simulink model "Gesamtsystem_Prototyp25_01_3"  (R2021b)
settings: Solver=FixedStepDiscrete  StartTime=0.0  StopTime=Inf  RelTol=1e-3  EnableMultiTasking=on
undefined symbols (not defined in the file): Down, GPTRIP1SEL, GPTRIP2SEL, magnitude, TZ1, TZ2, Up
libraries: c2837xDlib x18, hdlsllib x10, simulink x5, c2802xlib x5, c280xlib x3, dspsigops x3, commsequence2 x2, idelinklib_common x2, mcbcontrolslib x2, c2000lib x1, dspstat3 x1
(part 3 of 3)

== system Gesamtsystem_Prototyp25_01_3/Kommunikation/I2C Receiver/DecodeNexonar/Subsystem2 ==
  packed : Inport
  Bit Shift : hdlsllib/Logic and Bit Operations/Bit Shift  mode=Shift Left Logical  N=8
  Data Type Conversion : DataTypeConversion  OutDataTypeStr=int16
  Demux : Demux  Outputs=2
  Sum : Sum  Inputs=|++
  unpacked : Outport
  wires:
  packed/1 -> Demux/1
  Sum/1 -> Data Type Conversion/1
  Demux/1 -> Bit Shift/1
  Bit Shift/1 -> Sum/1
  Demux/2 -> Sum/2
  Data Type Conversion/1 -> unpacked/1

== system Gesamtsystem_Prototyp25_01_3/Kommunikation/I2C Receiver/DecodeNexonar/Subsystem3 ==
  packed : Inport
  Bit Shift : hdlsllib/Logic and Bit Operations/Bit Shift  mode=Shift Left Logical  N=8
  Data Type Conversion : DataTypeConversion  OutDataTypeStr=int16
  Demux : Demux  Outputs=2
  Sum : Sum  Inputs=|++
  unpacked : Outport
  wires:
  Data Type Conversion/1 -> unpacked/1
  Demux/2 -> Sum/2
  Bit Shift/1 -> Sum/1
  Demux/1 -> Bit Shift/1
  Sum/1 -> Data Type Conversion/1
  packed/1 -> Demux/1

== system Gesamtsystem_Prototyp25_01_3/Navigation und Uebergabe/Steuerung Fahrzeug/PWM/Drossel fuer Rueckwaertsfahren ==
  pwm_out_strecke : Inport
  rueckwaerts : Inport  Port=2
  Gain : Gain  Gain=0.8
  Switch : Switch  Criteria=u2 > Threshold
  Out1 : Outport
  wires:
  Gain/1 -> Switch/3
  rueckwaerts/1 -> Switch/2
  Switch/1 -> Out1/1
  pwm_out_strecke/1 -> Switch/1, Gain/1

== system Gesamtsystem_Prototyp25_01_3/Navigation und Uebergabe/Steuerung Fahrzeug/PWM/Drossel fuer Rueckwaertsfahren1 ==
  pwm_out_strecke : Inport
  rueckwaerts : Inport  Port=2
  Gain : Gain  Gain=0.8
  Switch : Switch  Criteria=u2 > Threshold
  Out1 : Outport
  wires:
  Gain/1 -> Switch/3
  rueckwaerts/1 -> Switch/2
  Switch/1 -> Out1/1
  pwm_out_strecke/1 -> Switch/1, Gain/1

== system Gesamtsystem_Prototyp25_01_3/Navigation und Uebergabe/Steuerung Fahrzeug/PWM/Inverter ==
  In1 : Inport
  Constant2 : Constant  Value=0
  Constant3 : Constant
  Switch : Switch  Criteria=u2 > Threshold  Threshold=0.5
  Out1 : Outport
  wires:
  Constant2/1 -> Switch/1
  Constant3/1 -> Switch/3
  In1/1 -> Switch/2
  Switch/1 -> Out1/1

== system Gesamtsystem_Prototyp25_01_3/Navigation und Uebergabe/Steuerung Fahrzeug/PWM/P-Regler mit Regelfehler Begrenzung Initial: k = 0.1, limit = +//- 100 Sampletime 0.1 ==
  a_soll : Inport
  a_ist : Inport  Port=2
  Abs : Abs  SampleTime=0.01
  Begrenzung : Saturate  UpperLimit=40  LowerLimit=0
  Betrag : MATLAB Function  TreatAsAtomicUnit=on  SystemSampleTime=0.01
  Dead Zone : DeadZone  LowerValue=-5  UpperValue=5  SaturateOnIntegerOverflow=on
  Richtung : MATLAB Function  TreatAsAtomicUnit=on  SystemSampleTime=0.01
  Sum : Sum  Inputs=|-+  SampleTime=0.01
  Verstaerkung : Gain  SampleTime=0.01
  pwm_out_a : Outport  VectorParamsAs1DForOutWhenUnconnected=off
  r/l_out_a : Outport  Port=2  VectorParamsAs1DForOutWhenUnconnected=off
  wires:
  Betrag/1(y) -> pwm_out_a/1
  Verstaerkung/1 -> Abs/1, Richtung/1(u)
  Sum/1 -> Dead Zone/1
  Abs/1 -> Begrenzung/1
  a_soll/1 -> Sum/2
  Richtung/1(y) -> r/l_out_a/1
  a_ist/1 -> Sum/1
  Begrenzung/1 -> Betrag/1(u)
  Dead Zone/1 -> Verstaerkung/1

== system Gesamtsystem_Prototyp25_01_3/Navigation und Uebergabe/Steuerung Fahrzeug/PWM/P-Regler mit Regelfehler Begrenzung Initial: k = 0.1, limit = +//- 100 Sampletime 0.2 ==
  strecke_ist : Inport
  strecke_soll : Inport  Port=2
  Abs : Abs  SampleTime=0.01
  Begrenzung : Saturate  UpperLimit=60  LowerLimit=0
  Betrag : MATLAB Function  TreatAsAtomicUnit=on  SystemSampleTime=0.01
  Dead Zone : DeadZone  SaturateOnIntegerOverflow=on
  Richtung : MATLAB Function  TreatAsAtomicUnit=on  SystemSampleTime=0.01
  Sum : Sum  Inputs=|-+  SampleTime=0.01
  Verstaerkung : Gain  Gain=1.5  SampleTime=0.01
  pwm_out_strecke : Outport  VectorParamsAs1DForOutWhenUnconnected=off
  r/l_out_strecke : Outport  Port=2  VectorParamsAs1DForOutWhenUnconnected=off
  wires:
  Betrag/1(y) -> pwm_out_strecke/1
  Verstaerkung/1 -> Abs/1, Richtung/1(u)
  Sum/1 -> Dead Zone/1
  Abs/1 -> Begrenzung/1
  strecke_soll/1 -> Sum/2
  Richtung/1(y) -> r/l_out_strecke/1
  strecke_ist/1 -> Sum/1
  Begrenzung/1 -> Betrag/1(u)
  Dead Zone/1 -> Verstaerkung/1

== matlab function Gesamtsystem_Prototyp25_01_3/Navigation und Uebergabe/Steuerung Fahrzeug/PWM/P-Regler mit Regelfehler Begrenzung Initial: k = 0.1, limit = +//- 100 Sampletime 0.1/Betrag ==
  settings: updateMethod=DISCRETE  sampleTime=0.01
  data: u input; y output
function y = fcn( u )

if u > 0.5
    y = u;
else
    y = 0;
end

== matlab function Gesamtsystem_Prototyp25_01_3/Navigation und Uebergabe/Steuerung Fahrzeug/PWM/P-Regler mit Regelfehler Begrenzung Initial: k = 0.1, limit = +//- 100 Sampletime 0.1/Richtung ==
  settings: updateMethod=DISCRETE  sampleTime=0.01
  data: u input; y output
function y = fcn( u )

if u > 0
    y = 1;
else
    y = 0;
end

== stateflow chart Gesamtsystem_Prototyp25_01_3/Navigation und Uebergabe/Steuerung Fahrzeug/PWM/Richtungsvorgabe links ==
  state Richtung_R
    r_l_out = r_l_out_strecke
  state Richtung_L
    r_l_out = r_l_out_a;
  (default) -> Richtung_R
  Richtung_R -> Richtung_L : [pwm_out_strecke < pwm_out_a]
  Richtung_L -> Richtung_R : [pwm_out_strecke >= pwm_out_a]
  data: r_l_out_strecke input; r_l_out_a input; pwm_out_strecke input; pwm_out_a input; r_l_out output

== stateflow chart Gesamtsystem_Prototyp25_01_3/Navigation und Uebergabe/Steuerung Fahrzeug/PWM/Stärke PWM L//R ==
  state a
    pwm_res_r = pwm_out_strecke + pwm_out_a;
    pwm_res_l = abs(pwm_out_strecke - pwm_out_a);
  state a1
    pwm_res_r = abs(pwm_out_strecke - pwm_out_a);
    pwm_res_l = pwm_out_strecke + pwm_out_a;
  (default) -> a
  a -> a1 : [r_l_out_a ~= r_l_out_strecke]
  a1 -> a : [r_l_out_a == r_l_out_strecke]
  data: r_l_out_a input; pwm_res_l output; r_l_out_strecke input; pwm_out_strecke input; pwm_out_a input; pwm_res_r output

== stateflow chart Gesamtsystem_Prototyp25_01_3/Navigation und Uebergabe/Steuerung Fahrzeug/PWM/Richtungsvorgabe rechts ==
  state Richtung_R
    r_l_out = r_l_out_strecke;
  state Richtung_L
    r_l_out = r_l_out_a;
  (default) -> Richtung_R
  Richtung_R -> Richtung_L : [pwm_out_strecke < pwm_out_a]
  Richtung_L -> Richtung_R : [pwm_out_strecke >= pwm_out_a]
  data: r_l_out_strecke input; r_l_out_a input; pwm_out_strecke input; pwm_out_a input; r_l_out output

== matlab function Gesamtsystem_Prototyp25_01_3/Navigation und Uebergabe/Steuerung Fahrzeug/PWM/P-Regler mit Regelfehler Begrenzung Initial: k = 0.1, limit = +//- 100 Sampletime 0.2/Betrag ==
  settings: updateMethod=DISCRETE  sampleTime=0.01
  data: u input; y output
function y = fcn( u )

if u > 0.5
    y = u;
else
    y = 0;
end

== matlab function Gesamtsystem_Prototyp25_01_3/Navigation und Uebergabe/Steuerung Fahrzeug/PWM/P-Regler mit Regelfehler Begrenzung Initial: k = 0.1, limit = +//- 100 Sampletime 0.2/Richtung ==
  settings: updateMethod=DISCRETE  sampleTime=0.01
  data: u input; y output
function y = fcn( u )

if u > 0
    y = 1;
else
    y = 0;
end

== matlab function Gesamtsystem_Prototyp25_01_3/Navigation und Uebergabe/Abwurf und Uebergabe/P-Regler mit Regelfehler Begrenzung Initial: k = 0.1, limit = +//- 100 Sampletime 0.1/Betrag ==
  settings: updateMethod=DISCRETE  sampleTime=0.01
  data: u input; y output
function y = fcn( u )

if u > 0.5
    y = u;
else
    y = 0;
end

== matlab function Gesamtsystem_Prototyp25_01_3/Navigation und Uebergabe/Abwurf und Uebergabe/P-Regler mit Regelfehler Begrenzung Initial: k = 0.1, limit = +//- 100 Sampletime 0.1/Richtung ==
  settings: updateMethod=DISCRETE  sampleTime=0.01
  data: u input; y output
function y = fcn( u )

if u > 0
    y = 1;
else
    y = 0;
end

== matlab function Gesamtsystem_Prototyp25_01_3/Navigation und Uebergabe/Abwurf und Uebergabe/P-Regler mit Regelfehler Begrenzung Initial: k = 0.1, limit = +//- 100 Sampletime 0.2/Betrag ==
  settings: updateMethod=DISCRETE  sampleTime=0.01
  data: u input; y output
function y = fcn( u )

if u > 0.5
    y = u;
else
    y = 0;
end

== matlab function Gesamtsystem_Prototyp25_01_3/Navigation und Uebergabe/Abwurf und Uebergabe/P-Regler mit Regelfehler Begrenzung Initial: k = 0.1, limit = +//- 100 Sampletime 0.2/Richtung ==
  settings: updateMethod=DISCRETE  sampleTime=0.01
  data: u input; y output
function y = fcn( u )

if u > 0
    y = 1;
else
    y = 0;
end

== stateflow chart Gesamtsystem_Prototyp25_01_3/Navigation und Uebergabe/Abwurf und Uebergabe/Abgabe_S_R_B ==
  state Abwurf_S
    y_soll_s = 100;
  state Stillstand
    y_ist_s = 0;
    y_ist_rb = 0;
    y_soll_rb = 0;
    y_soll_s = 0;
  state Abgabe_R_B
    y_soll_rb = 100;
    y_ist_rb = 100 - rb_dir*100;
  (default) -> Stillstand
  Stillstand -> Abgabe_R_B [order 1] : [rb == 1]
  Abwurf_S -> Stillstand : [s==0]
  Abgabe_R_B -> Stillstand : [rb == 0]
  Stillstand -> Abwurf_S [order 2] : [s==1]
  data: y_soll_rb output; y_ist_s output; y_ist_rb output; y_soll_s output; rb input; s input; rb_dir input

== stateflow chart Gesamtsystem_Prototyp25_01_3/Datenuebertragung zu stehendem System/Board Communication ==
  state Start
    n_rot = r;
    n_blau = b;
    andocken = 0;
    abdocken = 0;
    fin = 0;
    a = 0;
  state Andocking
    andocken = 1;
    abdocken = 0;
    a = 1;
  state Angedockt
  state Uebaergabe
    n_rot = r;
    n_blau = b;
    andocken = 1;
    abdocken = 0;
    a = 2;
  state Abdocken
    andocken = 0;
    abdocken = 1;
    a = 3;
  (default) -> Start
  Start -> Start [order 2] : after(0.5, sec)
  Uebaergabe -> Abdocken [order 1] : [zustand == 3]
  Angedockt -> Uebaergabe [order 2] : [zustand == 2]
  Start -> Andocking [order 1] : [zustand == 1]
  Andocking -> Angedockt : [andock == true ]
  Uebaergabe -> Abdocken [order 2] : after(15, sec)
  Angedockt -> Uebaergabe [order 1] : after(15, sec)
  data: n_rot output uint16; a output; andocken output; abdocken output; n_blau output uint16; fin output; b input uint16; r input uint16; zustand input; andock input

== stateflow chart Gesamtsystem_Prototyp25_01_3/Sortierung/Entscheidungen je nach Block ==
  state Roter_Block
    rot = 1;
    blau = 0;
    schwarz = 0;
  state Spannungsparameter_Berechnen
    grenze_rb = (u_rot + u_blau)/2;
    grenze_bs = (u_blau + u_schwarz)/2;
    rot_oben = grenze_rb -(u_blau - u_rot)/4;
    blau_unten = grenze_rb +(u_blau - u_rot)/4;
    blau_oben = grenze_bs - (u_schwarz - u_blau)/4;
    schwarz_unten = grenze_bs + (u_schwarz - u_blau)/4;
    init_farbe = 1;
    led_gruen = 0;
  state Roter_block
    u_rot = U_digital;
    led_rot = 0;
    led_gruen = 1;
  state blauer_block
    u_blau = U_digital;
  state schwarzer_block
    u_schwarz = U_digital;
  state Kontrollpunkt
    init_farbe = 0;
  state Zweites_Eingangsspannung
    U_in_2 = U_digital;
    block_2 = farbe(U_in_2, rot_oben, blau_unten, blau_oben, schwarz_unten);
  state Blauer_Block
    rot = 0;
    blau = 1;
    schwarz = 0;
  state grueneLED_zeichen
    led_gruen = 1;
  state grueneLED_zeichen1
    led_gruen = 0;
  state grueneLED_zeichen2
    led_gruen = 1;
  state Erstes_Eingangssignal
    U_in_1 = U_digital;
    block_1 = farbe(U_in_1, rot_oben, blau_unten, blau_oben, schwarz_unten);
  state Schwarzer_Block
    rot = 0;
    blau = 0;
    schwarz = 1;
  state Init_fehlgeschlagen
    led_rot = 1;
  Roter_Block -> Erstes_Eingangssignal : [U_digital >= 0.6]
  Zweites_Eingangsspannung -> Roter_Block [order 1] : [block_1 == 0 && block_2 == 0]
  Zweites_Eingangsspannung -> Erstes_Eingangssignal [order 4] : [block_1 ~= block_2]
  (default) -> Roter_block
  Kontrollpunkt -> Spannungsparameter_Berechnen [order 1] : [u_rot < u_blau && u_blau < u_schwarz]
  schwarzer_block -> Kontrollpunkt : [trigger3 == 1]
  Roter_block -> blauer_block : [trigger1 == 1]
  blauer_block -> schwarzer_block : [trigger2 == 1]
  Erstes_Eingangssignal -> Zweites_Eingangsspannung [order 1] : after(0.2, sec)
  grueneLED_zeichen1 -> grueneLED_zeichen2 : after(0.5, sec)
  grueneLED_zeichen2 -> Erstes_Eingangssignal : [bereit == 1]
  Zweites_Eingangsspannung -> Blauer_Block [order 2] : [block_1 ==1 && block_2 ==1]
  Spannungsparameter_Berechnen -> grueneLED_zeichen : after(0.5, sec)
  grueneLED_zeichen -> grueneLED_zeichen1 : after(0.5, sec)
  Blauer_Block -> Erstes_Eingangssignal : [U_digital <= 1.3 || U_digital >= 1.9]
  Kontrollpunkt -> Init_fehlgeschlagen [order 2] : [u_rot >= u_blau || u_blau >= u_schwarz || u_rot >= u_schwarz]
  Erstes_Eingangssignal -> Init_fehlgeschlagen [order 2] : [fertig_sortiert == 1]
  Schwarzer_Block -> Erstes_Eingangssignal : [U_digital < 2.0 || U_digital >= 2.6]
  Zweites_Eingangsspannung -> Erstes_Eingangssignal [order 5] : [block_1 == 3 || block_2 == 3]
  Zweites_Eingangsspannung -> Init_fehlgeschlagen [order 6] : [fertig_sortiert == 1]
  Zweites_Eingangsspannung -> Schwarzer_Block [order 3] : [block_1 == 2 && block_2 == 2]
  Init_fehlgeschlagen -> Roter_block : after(1, sec)
  data: U function_input; block function_output; rot_o function_input; blau_u function_input; blau_o function_input; schwarz_u function_input; fertig_sortiert input; led_gruen output; trigger1 input; trigger3 input; trigger2 input; led_rot output; bereit input; rot output; schwarz output; blau output; U_digital input; U_in local; U_in_2 local; block_2 local; block_1 local; U_in_1 local; init_farbe output; init_arr local; init_array local; u_blau local; u_schwarz local; u_rot local; grenze_bs local; grenze_rb local; rot_oben local; blau_unten local; blau_oben local; schwarz_unten local
  function block = farbe(U, rot_o, blau_u, blau_o, schwarz_u):
    | function block = farbe(U, rot_o, blau_u, blau_o, schwarz_u)
    |  if U < rot_o
    |      block = 0;
    |  elseif U > blau_u && U < blau_o
    |      block = 1;
    |  elseif U > schwarz_u && U < 3.0
    |      block = 2;
    |  else 
    |      block = 3;
    |  end

== stateflow chart Gesamtsystem_Prototyp25_01_3/Sortierung/Sortierscheibe/Auslenkung des Sortierrades ==
  state Grundzustand6
    n_rot = n_rot;
    schwarz  =1;
    rot = 0; duty = 1;
  state Grundzustand
    n_rot = i + 1;
    schwarz = 0;
    rot = 1; duty = 1;
  state Grundzustand3
    n_blau = j + 1;
  state Vorgaenger_blau
    auslenkung_soll = auslenkung_aktuell + 70;
  state drehen_entgegengesetzt1
    auslenkung_soll = auslenkung_aktuell - 70;
  state Vorgaenger_blau1
    auslenkung_soll = auslenkung_aktuell + 70;
  state Vorgaenger_rot_schwarz1
    auslenkung_soll = auslenkung_aktuell - 70;
  state Vorgaenger_rot_schwarz
    auslenkung_soll = auslenkung_aktuell - 70;
  state drehen_entgegengesetzt7
    auslenkung_soll = auslenkung_aktuell - 70;
  state drehen_entgegengesetzt8
    auslenkung_soll = auslenkung_aktuell + 70;
  state drehen_entgegengesetzt
    auslenkung_soll = auslenkung_aktuell + 70;
  state Warten2
    auslenkung_soll = auslenkung_ist;
    duty = 0;
  state Warten1
    auslenkung_soll = auslenkung_ist
    auslenkung_aktuell = auslenkung_ist;
  state Warten3
    auslenkung_soll = auslenkung_ist;
  state drehen_entgegengesetzt6
    auslenkung_soll = auslenkung_aktuell - 70;
  state Warten6
    auslenkung_soll = auslenkung_ist;
  state Auslenkung_blau
    auslenkung_soll = auslenkung_aktuell-70;
    j = n_blau; rs = 0; b = 1;
  state drehen_entgegengesetzt3
    auslenkung_soll = auslenkung_aktuell + 70;
  state Auslenkung_rotschwarz_vorgaenger1
    auslenkung_soll = auslenkung_aktuell+70;
    duty = 0; i = n_rot; rs = 1; b = 0;
  state Grundzustand2
    auslenkung_soll = auslenkung_aktuell-70;
    n_blau = 1;
  state Warten
    auslenkung_soll = auslenkung_ist;
    auslenkung_aktuell = auslenkung_ist;
  state drehen_entgegengesetzt2
    auslenkung_soll = auslenkung_aktuell + 70;
  state Grundzustand5
    auslenkung_soll = auslenkung_aktuell-70;
    n_rot = 0;
    schwarz = 1; duty = 1;
  state Grundzustand1
    auslenkung_soll = auslenkung_aktuell-70;
    n_rot = 1;
    rot = 1; duty = 1;
  state drehen_entgegengesetzt5
    auslenkung_soll = auslenkung_aktuell + 70;
  state drehen_entgegengesetzt4
    auslenkung_soll = auslenkung_aktuell + 70;
  state Warten5
    auslenkung_soll = auslenkung_ist;
    rs = 1; b = 0;
  state Warten4
    auslenkung_soll = auslenkung_ist;
    auslenkung_aktuell = auslenkung_ist;
  state Anfangsauslenkung
    auslenkung_soll = 140;
  state Warten_Start
    auslenkung_soll = 70;
    n_blau = 0; n_rot = 0;
    rot = 0; schwarz = 0; duty = 0;
  state Warten7
    auslenkung_soll = auslenkung_ist;
  state Stillstand
    auslenkung_soll = 0;
    duty = 0;
    n_blau = 0; n_rot = 0;
    schwarz = 0; rot = 0;
  Warten3 -> Grundzustand6 [order 3] : [Block_angekommen == 0 && blau == 0 && pos == 1]
  Warten3 -> Grundzustand3 [order 2] : [Block_angekommen == 0 && blau== 1]
  Warten3 -> Grundzustand [order 1] : [Block_angekommen == 0 && blau == 0 && pos == 0]
  Grundzustand -> Vorgaenger_blau1 [order 2] : [b == 1]
  Grundzustand -> Vorgaenger_rot_schwarz1 [order 1] : [rs == 1]
  Grundzustand6 -> Vorgaenger_blau1 [order 2] : [b == 1]
  Grundzustand6 -> Vorgaenger_rot_schwarz1 [order 1] : [rs == 1]
  Grundzustand3 -> Vorgaenger_rot_schwarz [order 1] : [rs == 1]
  Grundzustand3 -> Vorgaenger_blau [order 2] : [b == 1]
  Vorgaenger_blau -> drehen_entgegengesetzt1 [order 2] : after(1, sec)
  Vorgaenger_blau1 -> drehen_entgegengesetzt7 [order 2] : after(1, sec)
  drehen_entgegengesetzt8 -> Vorgaenger_rot_schwarz1 : [after(0.3, sec) || sortierscheibe_trigger == 0]
  drehen_entgegengesetzt -> Vorgaenger_rot_schwarz : [after(0.3, sec) || sortierscheibe_trigger == 0]
  Vorgaenger_rot_schwarz1 -> drehen_entgegengesetzt8 [order 2] : after(1, sec)
  drehen_entgegengesetzt1 -> Vorgaenger_blau : [after(0.3, sec) || sortierscheibe_trigger == 0]
  drehen_entgegengesetzt7 -> Vorgaenger_blau1 : [after(0.3, sec) || sortierscheibe_trigger == 0]
  Vorgaenger_rot_schwarz -> drehen_entgegengesetzt [order 2] : after(1, sec)
  Vorgaenger_blau -> Warten1 [order 1] : [abs(auslenkung_soll -auslenkung_ist) <5 && sortierscheibe_trigger == 0]
  Vorgaenger_rot_schwarz -> Warten1 [order 1] : [abs(auslenkung_soll -auslenkung_ist) <5 && sortierscheibe_trigger == 0]
  Vorgaenger_blau1 -> Warten2 [order 1] : [abs(auslenkung_soll -auslenkung_ist) <5 && sortierscheibe_trigger == 0]
  Vorgaenger_rot_schwarz1 -> Warten2 [order 1] : [abs(auslenkung_soll -auslenkung_ist) <5 && sortierscheibe_trigger == 0]
  Grundzustand1 -> Warten2 [order 1] : [abs(auslenkung_soll - auslenkung_ist) < 5 && sortierscheibe_trigger == 0]
  Grundzustand5 -> Warten2 [order 1] : [abs(auslenkung_soll - auslenkung_ist) < 5 && sortierscheibe_trigger == 0]
  Warten2 -> Auslenkung_rotschwarz_vorgaenger1 : after(0.75, sec)
  Grundzustand2 -> Warten1 [order 1] : [abs(auslenkung_soll - auslenkung_ist) < 5 && sortierscheibe_trigger == 0]
  Warten1 -> Auslenkung_blau : after(0.75, sec)
  Warten6 -> Warten3 : after(1, sec)
  drehen_entgegengesetzt6 -> Auslenkung_rotschwarz_vorgaenger1 : [after(0.3, sec) || sortierscheibe_trigger == 0]
  Auslenkung_rotschwarz_vorgaenger1 -> drehen_entgegengesetzt6 [order 2] : after(1, sec)
  Auslenkung_blau -> drehen_entgegengesetzt3 [order 2] : after(1, sec)
  drehen_entgegengesetzt3 -> Auslenkung_blau : [after(0.3, sec) || sortierscheibe_trigger == 0]
  Auslenkung_blau -> Warten [order 1] : [abs(auslenkung_soll - auslenkung_ist) < 5 && sortierscheibe_trigger == 0]
  Warten -> Warten6 : [Block_angekommen ==0]
  Auslenkung_rotschwarz_vorgaenger1 -> Warten [order 1] : [abs(auslenkung_soll - auslenkung_ist) < 5 && sortierscheibe_trigger == 0]
  drehen_entgegengesetzt2 -> Grundzustand2 : [after(0.3, sec) || sortierscheibe_trigger == 0]
  drehen_entgegengesetzt5 -> Grundzustand1 : [after(0.3, sec) || sortierscheibe_trigger == 0]
  Grundzustand5 -> drehen_entgegengesetzt4 [order 2] : after(1, sec)
  Grundzustand2 -> drehen_entgegengesetzt2 [order 2] : after(1, sec)
  Grundzustand1 -> drehen_entgegengesetzt5 [order 2] : after(1, sec)
  drehen_entgegengesetzt4 -> Grundzustand5 : [after(0.3, sec) || sortierscheibe_trigger == 0]
  Warten5 -> Grundzustand2 [order 1] : [Block_angekommen == 0 && blau== 1]
  Warten5 -> Grundzustand5 [order 3] : [Block_angekommen == 0 && blau == 0 && pos == 1]
  Warten5 -> Grundzustand1 [order 2] : [Block_angekommen == 0 && blau == 0 && pos == 0]
  Warten4 -> Warten5 : after(2, sec)
  Anfangsauslenkung -> Warten4 : [Block_angekommen == 0]
  Warten_Start -> Anfangsauslenkung : after(7, sec)
  Warten7 -> Warten_Start : after(4, sec)
  Stillstand -> Warten7 : [init_farbe == 1]
  (default) -> Stillstand
  data: sortierscheibe_trigger input; n_rot output uint16; duty output; rot output; n_blau output uint16; auslenkung_soll output; Block_angekommen input; auslenkung_ist input; blau input; pos input; i local uint16; j local uint16; schwarz output; init_farbe input; auslenkung_aktuell local; rs local; b local

== matlab function Gesamtsystem_Prototyp25_01_3/Sortierung/Sortierscheibe/P-Regler mit Regelfehler Begrenzung Initial: k = 0.1, limit = +//- 100 Sampletime 0.1/Betrag ==
  settings: updateMethod=DISCRETE  sampleTime=0.01
  data: u input; y output
function y = fcn( u )

if u > 0.5
    y = u;
else
    y = 0;
end

== matlab function Gesamtsystem_Prototyp25_01_3/Sortierung/Sortierscheibe/P-Regler mit Regelfehler Begrenzung Initial: k = 0.1, limit = +//- 100 Sampletime 0.1/Richtung ==
  settings: updateMethod=DISCRETE  sampleTime=0.01
  data: u input; y output
function y = fcn( u )

if u > 0
    y = 1;
else
    y = 0;
end

== stateflow chart Gesamtsystem_Prototyp25_01_3/Sortierung/Weiche/Motor Weiche steuerung ==
  note: pos ist 0 wenn auf rot gestellt
  state Bewegung_nach_rot
    pos=0;
  state Bewegung_nach_blau
    pos=1;
  (default) -> Bewegung_nach_rot
  Bewegung_nach_blau -> Bewegung_nach_rot : [work == 1 && rot == 1 && schwarz == 0]
  Bewegung_nach_rot -> Bewegung_nach_blau : [work == 1 && rot == 0 && schwarz == 1]
  data: rot input; schwarz input; work input; pos output

== matlab function Gesamtsystem_Prototyp25_01_3/Kommunikation/I2C Reset (behebt Stabilitätsprobleme der I2C-Verbindung)/I2C Reset/I2C Reset ==
function fcn()
%#codegen

coder.ceval( 'reset_i2c' );

== stateflow chart Gesamtsystem_Prototyp25_01_3/Sortierung/Weiche/Motor Weiche steuerung1 ==
  state Startausrichtung
    y_soll= y_start;
    y_soll_n = 0;
    pos = 0;
  note: pos ist 0 wenn auf rot gestellt
  state Bewegung_nach_rot
    y_soll =0;
    y_soll_n = y_rot;
    pos = 0;
  state Bereit
    y_soll = 0;
    y_soll_n = 0;
  state Bewegung_nach_schwarz
    y_soll = y_blau;
    y_soll_n = 0;
    pos = 1;
  state Warten
    y_soll = 0;
    y_soll_n = 0;
  state Warten1
    y_soll = 0;
    y_soll_n = 0;
  (default) -> Startausrichtung
  Startausrichtung -> Bereit : after(0.5, sec)
  Bereit -> Bewegung_nach_schwarz [order 2] : [duty == 1 && schwarz == 1 && rot == 0 && pos == 0]
  Bereit -> Bewegung_nach_rot [order 1] : [duty == 1 && schwarz == 0 && rot == 1 && pos == 1]
  Warten -> Bereit
  Warten1 -> Bereit
  Bewegung_nach_rot -> Warten : after(0.2, sec)
  Bewegung_nach_schwarz -> Warten1 : after(0.2, sec)
  data: rot input; schwarz input; work input; y_soll_n output; y_soll output; y_start input; y_rot input; y_blau input; duty input; pos local

== matlab function Gesamtsystem_Prototyp25_01_3/Sortierung/Weiche/P-Regler mit Regelfehler Begrenzung Initial: k = 0.1, limit = +//- 100 Sampletime 0.01/Betrag ==
  settings: updateMethod=DISCRETE  sampleTime=0.01
  data: u input; y output
function y = fcn( u )

if u > 0.5
    y = u;
else
    y = 0;
end

== matlab function Gesamtsystem_Prototyp25_01_3/Kommunikation/I2C Reset (behebt Stabilitätsprobleme der I2C-Verbindung)/I2C Reinitialisierung/I2C Reinitialisierung ==
function fcn()
%#codegen

coder.ceval( 'init_i2c' );

== matlab function Gesamtsystem_Prototyp25_01_3/Sortierung/Weiche/P-Regler mit Regelfehler Begrenzung Initial: k = 0.1, limit = +//- 100 Sampletime 0.01/Richtung ==
  settings: updateMethod=DISCRETE  sampleTime=0.01
  data: u input; y output
function y = fcn( u )

if u > 0
    y = 1;
else
    y = 0;
end

== stateflow chart Gesamtsystem_Prototyp25_01_3/Navigation und Uebergabe/Fahrtrichtungsangaben1 ==
  state Init
    x_off = x_ist; y_off = y_ist; z_off = z_ist; a_off = a_ist;
    x_soll = x_ist, y_soll = y_ist;
    rueckwaerts = 1; steuerung = 0;
    anfahrt = 0;
    rb_dir=0; ende = 1;
    count1=0; count2 = 0;
    fertig_sortiert = 0;
  state Position5_lenkung
    x_soll = x_soll_array(1);
    y_soll = y_soll_array(1);
    steuerung = 1;
    a_soll = a_ziel(x_ist, x_soll, y_ist, y_soll);
    ende = 0;
  state Position5
    x_soll = x_soll_array(1);
    y_soll = y_soll_array(1);
    steuerung = 0;
  state Zwischenposition1_lenkung
    x_soll = x_soll_array(2);
    y_soll = y_soll_array(2);
    steuerung = 1;
    a_soll = a_ziel(x_ist,x_soll,y_ist,y_soll);
  state Zwischenposition1
    x_soll = x_soll_array(2);
    y_soll = y_soll_array(2);
    steuerung = 0;
  state Position3_lenkung
    x_soll = x_soll_array(3);
    y_soll = y_soll_array(3);
    steuerung = 1;
    a_soll = a_ziel(x_ist,x_soll,y_ist,y_soll);
  state Position3
    x_soll = x_soll_array(3);
    y_soll = y_soll_array(3);
    steuerung = 0;
  state Zwischenposition2_lenkung
    x_soll = x_soll_array(4);
    y_soll = y_soll_array(4);
    steuerung = 1;
    a_soll = a_ziel(x_ist,x_soll,y_ist,y_soll);
  state Zwischenposition2
    x_soll = x_soll_array(4);
    y_soll = y_soll_array(4);
    steuerung = 0;
  state Zwischenposition7_lenkung
    x_soll = x_soll_array(14)-2*(x_soll_array(14)-x_ist);
    y_soll = y_soll_array(14)-2*(y_soll_array(14)-y_ist);
    steuerung = 1;
    rueckwaerts = 0;
    a_soll = a_ziel(x_ist,x_soll,y_ist,y_soll);
  state Zwischenposition7
    x_soll = x_soll_array(14);
    y_soll = y_soll_array(14);
    steuerung = 0;
    rueckwaerts = 0;
  state Position4_lenkung
    x_soll = x_soll_array(5);
    y_soll = y_soll_array(5);
    steuerung = 1; rueckwaerts = 1;
    a_soll = a_ziel(x_ist,x_soll,y_ist,y_soll);
  state Position4
    x_soll = x_soll_array(5);
    y_soll = y_soll_array(5);
    steuerung = 0;
  state Zwischenposition3_lenkung
    x_soll = x_soll_array(6);
    y_soll = y_soll_array(6);
    steuerung = 1;
    a_soll = a_ziel(x_ist,x_soll,y_ist,y_soll);
  state Zwischenposition3
    x_soll = x_soll_array(6);
    y_soll = y_soll_array(6);
    steuerung = 0;
  state Zwischenposition8_lenkung
    x_soll = x_soll_array(15);
    y_soll = y_soll_array(15);
    steuerung = 1;
    a_soll = a_ziel(x_ist,x_soll,y_ist,y_soll);
  state Zwischenposition8
    x_soll = x_soll_array(15);
    y_soll = y_soll_array(15);
    steuerung  = 0;
  state Position2_lenkung
    x_soll = x_soll_array(7);
    y_soll = y_soll_array(7);
    steuerung = 1;
    a_soll = a_ziel(x_ist,x_soll,y_ist,y_soll);
  state Position2
    x_soll = x_soll_array(7);
    y_soll = y_soll_array(7);
    steuerung  = 0;
  state Zwischenposition4_lenkung
    x_soll = x_soll_array(8);
    y_soll = y_soll_array(8);
    steuerung = 1;
    a_soll = a_ziel(x_ist,x_soll,y_ist,y_soll);
  state Zwischenposition4
    x_soll = x_soll_array(8);
    y_soll = y_soll_array(8);
    steuerung = 0;
  state Warten
    x_soll = x_ist;
    y_soll = y_ist;
  state Position1_lenkung
    x_soll = x_soll_array(9);
    y_soll = y_soll_array(9);
    steuerung = 1;
    a_soll = a_ziel(x_ist,x_soll,y_ist,y_soll);
  state Andocken_lenkung
    x_soll = x_ist;
    y_soll = y_ist - 1000;
    rueckwaerts = 0;
    steuerung = 1;
    a_soll = a_ziel(x_ist,x_soll,y_ist,y_soll);
  state Zwischenposition5_lenkung
    x_soll = x_soll_array(10);
    y_soll = y_soll_array(10);
    steuerung = 1;
    a_soll = a_ziel(x_ist,x_soll,y_ist,y_soll);
    anfahrt = 1;
  state Zwischenposition5
    x_soll = x_soll_array(10);
    y_soll = y_soll_array(10);
    steuerung = 0;
  state Docked
    x_soll = x_ist;
    y_soll = y_ist;
    steuerung = 0;
    rueckwaerts = 1;
  state Position1
    x_soll = x_soll_array(9);
    y_soll = y_soll_array(9);
    steuerung = 0;
  state Andocken
    x_soll = x_ist;
    y_soll = y_ist - 1000;
    rueckwaerts = 0;
    steuerung = 0;
  state Uebergabe_Rot_Blau
    rb = 1;
    rb_dir=1;
    x_soll = x_ist;
    y_soll = y_ist;
    steuerung = 0;
    rueckwaerts = 1;
    count2 = count1 +1;
  state a = a_ziel(x_i,x_s,y_i,y_s) [function]
  state Uebergabe_Rot_Blau1
    rb = 1;
    rb_dir=(-1);
    x_soll = x_ist;
    y_soll = y_ist;
    steuerung = 0;
    rueckwaerts = 1;
    count1 = count2 + 1;
  state Uebergabe_Rot_Blau2
    rb = 0;
    rb_dir=0;
    x_soll = x_ist;
    y_soll = y_ist;
    steuerung = 0;
    rueckwaerts = 1;
  state Schwarz_Abwurf
    x_soll = x_ist;
    y_soll = y_ist-1000;
    steuerung = 0;
  state Schwarz_Abwurf_lenkung
    x_soll = x_ist;
    y_soll = y_ist+1000;
    steuerung = 1;
    rueckwaerts = 0;
    a_soll = a_ziel(x_ist,x_soll,y_ist,y_soll);
  state Stop
    x_soll = x_ist;
    y_soll = y_ist;
    ende = 1;
  state Zwischenposition6
    x_soll = x_soll_array(12);
    y_soll = y_soll_array(12);
    steuerung = 0;
  state Zwischenposition6_lenkung
    x_soll = x_soll_array(12);
    y_soll = y_soll_array(12);
    steuerung = 1;
    a_soll = a_ziel(x_ist,x_soll,y_ist,y_soll);
  state Rueckkehr
    x_soll = x_soll_array(10);
    y_soll = y_soll_array(10);
    steuerung = 0;
    fertig_sortiert = 1;
  state Abwurf_schwarz
    x_soll = x_ist;
    y_soll = y_ist;
    s = 0;
  state Stop_schwarz
    x_soll = x_ist;
    y_soll = y_ist;
    s = 1;
  Position5_lenkung -> Docked [order 2] : [andock == 1]
  (default) -> Init
  Position5 -> Docked [order 3] : [andock == 1]
  Init -> Position5_lenkung : [start == 1]
  Zwischenposition1_lenkung -> Docked [order 2] : [andock == 1]
  Position5 -> Position5_lenkung [order 2] : [abs(a_ist-a_soll) >=250]
  Position5_lenkung -> Position5 [order 1] : [abs(a_ist-a_soll) < 100]
  Zwischenposition1 -> Docked [order 3] : [andock == 1]
  Position5 -> Zwischenposition1_lenkung [order 1] : [abs(x_soll -x_ist)< 600 && abs(y_soll - y_ist)<600]
  Position3_lenkung -> Docked [order 2] : [andock == 1]
  Zwischenposition1 -> Zwischenposition1_lenkung [order 2] : [abs(a_ist-a_soll) >=250]
  Zwischenposition1_lenkung -> Zwischenposition1 [order 1] : [abs(a_ist-a_soll) < 100]
  Position3 -> Docked [order 2] : [andock == 1]
  Zwischenposition1 -> Position3_lenkung [order 1] : [abs(x_soll -x_ist)< 600 && abs(y_soll - y_ist)<600]
  Zwischenposition2_lenkung -> Docked [order 2] : [andock == 1]
  Position3 -> Position3_lenkung [order 1] : [abs(a_ist-a_soll) >=250]
  Position3_lenkung -> Position3 [order 1] : [abs(a_ist-a_soll) < 100]
  Zwischenposition2 -> Docked [order 2] : [andock == 1]
  Position3 -> Zwischenposition2_lenkung [order 3] : [abs(x_soll -x_ist)< 600 && abs(y_soll - y_ist)<600]
  Zwischenposition7_lenkung -> Docked [order 2] : [andock == 1]
  Zwischenposition2_lenkung -> Zwischenposition2 [order 1] : [abs(a_ist-a_soll) < 100]
  Zwischenposition2 -> Zwischenposition2_lenkung [order 1] : [abs(a_ist-a_soll) >=250]
  Zwischenposition7 -> Docked [order 2] : [andock == 1]
  Zwischenposition2 -> Zwischenposition7_lenkung [order 3] : [abs(x_soll -x_ist)< 600 && abs(y_soll - y_ist)<600]
  Zwischenposition7_lenkung -> Zwischenposition5_lenkung [order 3] : [timer == 1]
  Position4_lenkung -> Docked [order 2] : [andock == 1]
  Zwischenposition7_lenkung -> Zwischenposition7 [order 1] : [abs(a_ist-a_soll) < 100]
  Zwischenposition7 -> Zwischenposition7_lenkung [order 1] : [abs(a_ist-a_soll) >=250]
  Zwischenposition7 -> Zwischenposition5_lenkung [order 4] : [timer == 1]
  Position4 -> Docked [order 2] : [andock == 1]
  Zwischenposition7 -> Position4_lenkung [order 3] : [abs(x_soll -x_ist)< 600 && abs(y_soll - y_ist)<600]
  Zwischenposition3_lenkung -> Docked [order 2] : [andock == 1]
  Position4_lenkung -> Zwischenposition5_lenkung [order 3] : [timer == 1]
  Position4_lenkung -> Position4 [order 1] : [abs(a_ist-a_soll) < 50]
  Position4 -> Position4_lenkung [order 4] : [abs(a_ist-a_soll) >=250]
  Position4 -> Zwischenposition5_lenkung [order 1] : [timer == 1]
  Position4 -> Zwischenposition3_lenkung [order 3] : [abs(x_soll -x_ist)< 600 && abs(y_soll - y_ist)<600]
  Zwischenposition3 -> Docked [order 2] : [andock == 1]
  Zwischenposition3_lenkung -> Zwischenposition5_lenkung [order 3] : [timer == 1]
  Zwischenposition3_lenkung -> Zwischenposition3 [order 1] : [abs(a_ist-a_soll) < 100]
  Zwischenposition3 -> Zwischenposition3_lenkung [order 4] : [abs(a_ist-a_soll) >=250]
  Zwischenposition8_lenkung -> Docked [order 1] : [andock == 1]
  Zwischenposition3 -> Zwischenposition5_lenkung [order 1] : [timer == 1]
  Zwischenposition3 -> Zwischenposition8_lenkung [order 3] : [abs(x_soll -x_ist)< 600 && abs(y_soll - y_ist)<600]
  Zwischenposition8 -> Docked [order 2] : [andock == 1]
  Zwischenposition8_lenkung -> Zwischenposition5_lenkung [order 3] : [timer == 1]
  Zwischenposition8 -> Zwischenposition8_lenkung [order 1] : [abs(a_ist-a_soll) >=250]
  Zwischenposition8_lenkung -> Zwischenposition8 [order 2] : [abs(a_ist-a_soll) < 100]
  Position2_lenkung -> Docked [order 2] : [andock == 1]
  Zwischenposition8 -> Zwischenposition5_lenkung [order 3] : [timer == 1]
  Zwischenposition8 -> Position2_lenkung [order 4] : [abs(x_soll -x_ist)< 600 && abs(y_soll - y_ist)< 600]
  Position2 -> Docked [order 2] : [andock == 1]
  Position2_lenkung -> Zwischenposition5_lenkung [order 3] : [timer == 1]
  Zwischenposition4_lenkung -> Docked [order 2] : [andock == 1]
  Position2 -> Position2_lenkung [order 3] : [abs(a_ist-a_soll) >=250]
  Position2_lenkung -> Position2 [order 1] : [abs(a_ist-a_soll) < 100]
  Zwischenposition4 -> Docked [order 1] : [andock == 1]
  Position2 -> Zwischenposition5_lenkung [order 4] : [timer == 1]
  Position2 -> Zwischenposition4_lenkung [order 1] : [abs(x_soll -x_ist)< 600 && abs(y_soll - y_ist)< 600]
  Zwischenposition4_lenkung -> Zwischenposition5_lenkung [order 3] : [timer == 1]
  Zwischenposition4_lenkung -> Zwischenposition4 [order 1] : [abs(a_ist-a_soll) <100]
  Zwischenposition4 -> Zwischenposition4_lenkung [order 3] : [abs(a_ist-a_soll) >=250]
  Position1_lenkung -> Docked [order 2] : [andock == 1]
  Position1 -> Docked [order 2] : [andock == 1]
  Zwischenposition4 -> Zwischenposition5_lenkung [order 4] : [timer == 1]
  Zwischenposition4 -> Warten [order 2] : [abs(x_soll -x_ist)< 600 && abs(y_soll - y_ist)<600]
  Zwischenposition5_lenkung -> Docked [order 2] : [andock == 1]
  Warten -> Position1_lenkung : after(5, sec)
  Zwischenposition5 -> Docked [order 2] : [andock == 1]
  Andocken_lenkung -> Docked [order 1] : [andock == 1]
  Position1 -> Position1_lenkung [order 3] : [abs(a_ist-a_soll) >=250]
  Position1_lenkung -> Position1 [order 1] : [abs(a_ist-a_soll) < 100]
  Andocken -> Docked [order 2] : [andock == 1]
  Zwischenposition5 -> Zwischenposition5_lenkung [order 3] : [abs(a_ist-a_soll) >=250]
  Andocken_lenkung -> Andocken [order 2] : [abs(a_ist-a_soll) < 50]
  Zwischenposition5 -> Andocken_lenkung [order 1] : [x_ist >= x_soll]
  Position1 -> Zwischenposition5_lenkung [order 1] : [abs(x_soll -x_ist)< 600 && abs(y_soll - y_ist)<600]
  Andocken -> Andocken_lenkung [order 3] : [abs(a_ist-a_soll) >=150]
  Zwischenposition5_lenkung -> Zwischenposition5 [order 1] : [abs(a_ist-a_soll) < 100]
  Andocken -> Docked [order 1] : [abs(x_ist-x_soll) < 800 && abs(y_ist-y_soll)<800]
  Docked -> Uebergabe_Rot_Blau [order 2] : after(10, sec)
  Docked -> Uebergabe_Rot_Blau [order 1] : [zustand >= 2]
  Uebergabe_Rot_Blau -> Uebergabe_Rot_Blau1 : after(1.5, sec)
  Uebergabe_Rot_Blau1 -> Uebergabe_Rot_Blau [order 2] : after(1.5, sec)
  Uebergabe_Rot_Blau1 -> Uebergabe_Rot_Blau2 [order 1] : [count1>=4]
  Schwarz_Abwurf_lenkung -> Schwarz_Abwurf [order 1] : [abs(a_ist-a_soll) < 50]
  Rueckkehr -> Zwischenposition6_lenkung : [abs(y_soll - y_ist)<600]
  Zwischenposition6 -> Schwarz_Abwurf_lenkung [order 2] : [abs(x_ist-x_soll)<=600 && abs(y_ist - y_soll) <= 600]
  Uebergabe_Rot_Blau2 -> Rueckkehr [order 1] : [zustand == 3]
  Zwischenposition6_lenkung -> Zwischenposition6 : [abs(a_ist-a_soll) <50]
  Schwarz_Abwurf -> Schwarz_Abwurf_lenkung [order 1] : [abs(a_ist-a_soll) >=150]
  Zwischenposition6 -> Zwischenposition6_lenkung [order 1] : [abs(a_ist-a_soll) >=150]
  Uebergabe_Rot_Blau2 -> Rueckkehr [order 2] : after(10, sec)
  Abwurf_schwarz -> Stop : after(1, sec)
  Schwarz_Abwurf -> Stop_schwarz [order 2] : [y_ist < y_soll_array(13) || trigger == 0]
  Schwarz_Abwurf_lenkung -> Stop_schwarz [order 2] : [trigger == 0]
  Stop_schwarz -> Abwurf_schwarz : after(2, sec)
  data: x_i function_input double size=1; x_s function_input double size=1; y_i function_input double size=1; y_s function_input double size=1; a function_output double; trigger input; timer input; ende output; s output; rb output; andock input; start input; rueckwaerts output; x_ist input double; y_ist input double; a_ist input double; z_ist input double; x_off local double; z_off local double; a_off local double; y_off local double; x_soll output double; steuerung output; y_soll output double; x_in local double; y_in local double; fin local boolean; y_soll_array input double; x_soll_array input double; zustand input; andock_l input; andock_r input; anfahrt output; fertig_sortiert output; rb_dir output; count local; a_soll local double; count1 local; count2 local

== stateflow chart Gesamtsystem_Prototyp25_01_3/Navigation und Uebergabe/Positionsbestimmung1 ==
  state Position4
    x_soll_array(5)=x_ist+100;
    y_soll_array(5)=y_ist+400;
    x_soll_array(6)=x_ist+200;
    y_soll_array(6)=y_ist+650;
    x_soll_array(15)=x_ist-1000;
    y_soll_array(15)=y_ist+800;
  state Position3
    x_soll_array(3)=x_ist-150;
    y_soll_array(3)=y_ist-250;
    x_soll_array(4)=x_ist-500;
    y_soll_array(4)=y_ist+1000;
    x_soll_array(14)=x_ist+800;
    y_soll_array(14)=y_ist-1500;
  state Init
    x_soll_array = [14000, 10000, 8000, 8750, 9000, 9500, 5000, 3500, 3500, 14000, 14000, 8000, 8000, 9000, 8000];
    y_soll_array = [500, 1000, 4000, 5500, 7000, 8000, 8000, 8000, 2500, -500, 2500, 2500, -1500, 3000. 8000];
    init = 0;
    docked = false; ende = 0;
  state Position5
    x_soll_array(1)=x_ist;
    y_soll_array(1)=y_ist-400;
    x_soll_array(2)=x_ist-4000;
    y_soll_array(2)=y_ist+300;
  state Position2
    x_soll_array(7)=x_ist+600;
    y_soll_array(7)=y_ist-700;
    x_soll_array(8)=x_ist-1000;
    y_soll_array(8)=y_ist-800;
  state Notfall_Ende
    ende = 1;
  state Andocken
    x_soll_array(11)=x_ist;
    y_soll_array(11)=y_ist-300;
    x_soll_array(10)=x_ist;
    y_soll_array(10)=y_ist-2800;
  state Position1
    x_soll_array(9)=x_ist-100;
    y_soll_array(9)=y_ist+100;
  state Ziel
    x_soll_array(13)=x_ist-100;
    y_soll_array(13)=y_ist+300;
    x_soll_array(12)=x_ist;
    y_soll_array(12)=y_ist+3000;
  state Ende_Timer
    timer = 1;
  state Senden
    init = 1;
    timer = 0;
  state Fertig
  state Docked
    docked = true;
  (default) -> Init
  Position5 -> Position3 : [trigger ==0]
  Position4 -> Position2 : [trigger ==0]
  Position3 -> Position4 : [trigger ==1]
  Init -> Position5 : [trigger ==1]
  Position2 -> Position1 : [trigger ==1]
  Senden -> Notfall_Ende [order 3] : [trigger == 0]
  Andocken -> Ziel : [trigger ==1]
  Position1 -> Andocken : [trigger ==0]
  Ziel -> Fertig : [trigger ==0]
  Fertig -> Senden : [trigger == 1]
  Senden -> Ende_Timer [order 1] : after(100, sec)
  Docked -> Senden : [abs(x_ist-x_soll_array(11))>=400 && abs(y_ist-y_soll_array(11))>=800]
  Senden -> Docked [order 2] : [abs(x_ist-x_soll_array(11))<400 && abs(y_ist-y_soll_array(11))<800]
  data: docked output boolean; trigger input; x_ist input; y_ist input; x_soll_array output; timer output; init output; y_soll_array output; ende output
